simulink model "AE432_FinDel_Pioneer_WayPoint_Sim_2018a"  (R2018a)
settings: Solver=VariableStepAuto  StartTime=0  StopTime=445  FixedStep=T  RelTol=1e-3  EnableMultiTasking=on
InitFcn:
  | Waypoints
  | RollPitchTracking_Stab_ControlPioneer
values from neighbouring files (symbols this model uses):
  h = 220*ones(1,36)    [Waypoints.m]
  K1 = place(Along,Blong,P1)    [RollPitchTracking_Stab_ControlPioneer.m]
  T = 0.05    [Waypoints.m]
  x = [0 250 250 250 250 250 1250 2250 2150 2100 2050 2000 1900 1250 1250 500 500 500 500 1500 2250 2250 2250 2250 1000 1000 1000 1000 1250 1250 1250 1250 1750 1750 1750 1750]    [Waypoints.m]
  y = [0 1250 1750 2750 3500 4250 4250 4250 3750 3000 1750 1250 250 250 1500 2500 3000 3500 4000 4000 4000 3500 3000 2500 2500 3000 3500 4000 4000 3500 3000 2500 2500 3000 3500 4000]    [Waypoints.m]
undefined symbols (not defined in the file or in its folder): DiscIntNeverNeededParam, Td
libraries: simulink x19, simulink_extras x10, aerolibfltsims x2, airlib x1, aerolibanimutils x1
(part 2 of 2)

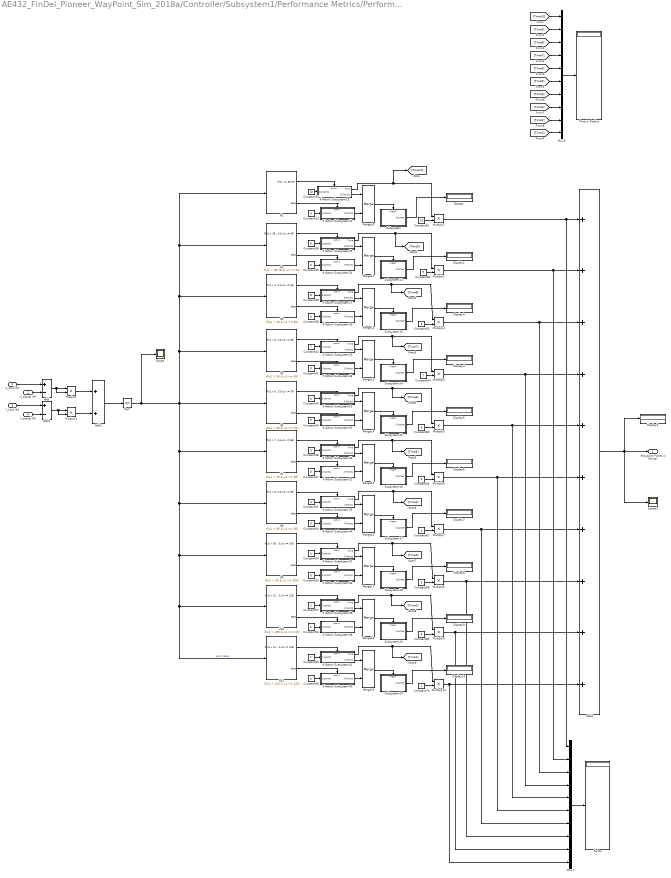
== system AE432_FinDel_Pioneer_WayPoint_Sim_2018a/Controller/Subsystem1/Performance Metrics/Performance Index Waypoints ==
  X_cmd (ft) : Inport
  X_actual (ft) : Inport  Port=2
  Y_cmd (ft) : Inport  Port=3
  Y_actual (ft) : Inport  Port=4
  Add : Sum  Inputs=+-
  Add1 : Sum  Inputs=+-
  Add2 : Sum
  Add4 : Sum  Inputs=10
  Constant{32,35,38,41,44,47,50,53,56,59} (10 alike) : Constant  Value=0
  Constant33 : Constant  Value=10
  Constant36 : Constant  Value=9
  Constant39 : Constant  Value=8
  Constant42 : Constant  Value=7
  Constant45 : Constant  Value=6
  Constant48 : Constant  Value=5
  Constant51 : Constant  Value=4
  Constant54 : Constant  Value=3
  Constant57 : Constant  Value=2
  Constant60 : Constant
  Constant61 : Constant  Value=10
  Constant62 : Constant  Value=9
  Constant63 : Constant  Value=8
  Constant64 : Constant  Value=7
  Constant65 : Constant  Value=6
  Constant66 : Constant  Value=5
  Constant67 : Constant  Value=4
  Constant68 : Constant  Value=3
  Constant69 : Constant  Value=2
  Constant70 : Constant
  Display{,1..10} (11 alike) : Display
  If Action Subsystem22 : Subsystem  TreatAsAtomicUnit=on
  If Action Subsystem23 : Subsystem  TreatAsAtomicUnit=on
  If Action Subsystem24 : Subsystem  TreatAsAtomicUnit=on
  If Action Subsystem25 : Subsystem  TreatAsAtomicUnit=on
  If Action Subsystem26 : Subsystem  TreatAsAtomicUnit=on
  If Action Subsystem27 : Subsystem  TreatAsAtomicUnit=on
  If Action Subsystem28 : Subsystem  TreatAsAtomicUnit=on
  If Action Subsystem29 : Subsystem  TreatAsAtomicUnit=on
  If Action Subsystem30 : Subsystem  TreatAsAtomicUnit=on
  If Action Subsystem31 : Subsystem  TreatAsAtomicUnit=on
  If Action Subsystem32 : Subsystem  TreatAsAtomicUnit=on
  If Action Subsystem33 : Subsystem  TreatAsAtomicUnit=on
  If Action Subsystem34 : Subsystem  TreatAsAtomicUnit=on
  If Action Subsystem35 : Subsystem  TreatAsAtomicUnit=on
  If Action Subsystem36 : Subsystem  TreatAsAtomicUnit=on
  If Action Subsystem37 : Subsystem  TreatAsAtomicUnit=on
  If Action Subsystem38 : Subsystem  TreatAsAtomicUnit=on
  If Action Subsystem39 : Subsystem  TreatAsAtomicUnit=on
  If Action Subsystem40 : Subsystem  TreatAsAtomicUnit=on
  If Action Subsystem41 : Subsystem  TreatAsAtomicUnit=on
  If10 : If  IfExpression=u1 > 105 & u1 <= 115
  If11 : If  IfExpression=u1 > 115 & u1 <= 125
  If2 : If  IfExpression=u1 <= 33.76
  If3 : If  IfExpression=u1 > 33.76 & u1 <= 45
  If4 : If  IfExpression=u1 > 45 & u1 <= 55
  If5 : If  IfExpression=u1 > 55 & u1 <= 65
  If6 : If  IfExpression=u1 > 65 & u1 <= 75
  If7 : If  IfExpression=u1 > 75 & u1 <= 85
  If8 : If  IfExpression=u1 > 85 & u1 <= 95
  If9 : If  IfExpression=u1 > 95 & u1 <= 105
  Merge{10..19} (10 alike) : Merge
  Multiply{1..10} (10 alike) : Product
  Mux1 : Mux  Inputs=10
  Mux2 : Mux  Inputs=10
  Points : Display
  Product : Product  RndMeth=Zero
  Product1 : Product  RndMeth=Zero
  Scope : Scope
  Scope2 : Scope
  Sqrt : Sqrt  SaturateOnIntegerOverflow=on
  Subsystem : Subsystem
  Subsystem12 : Subsystem
  Subsystem13 : Subsystem
  Subsystem14 : Subsystem
  Subsystem15 : Subsystem
  Subsystem16 : Subsystem
  Subsystem17 : Subsystem
  Subsystem18 : Subsystem
  Subsystem19 : Subsystem
  Subsystem20 : Subsystem
  Time in Radius : Display
  Waypoint Points = f(time) : Outport
  wires:
  Subsystem19/1(Counter) -> Display9/1
  Subsystem20/1(Counter) -> Display10/1
  Add/1 -> Product/2, Product/1
  Add1/1 -> Product1/2, Product1/1
  Y_actual (ft)/1 -> Add1/2
  Product1/1 -> Add2/2
  X_cmd (ft)/1 -> Add/1
  Product/1 -> Add2/1
  Y_cmd (ft)/1 -> Add1/1
  X_actual (ft)/1 -> Add/2
  Add2/1 -> Sqrt/1
  Sqrt/1 -> Scope/1, If11/1, If10/1, If9/1, If8/1, If7/1, If6/1, If5/1, If4/1, If3/1, If2/1  "error radius"
  If Action Subsystem22/1(0 Points) -> Merge10/2
  If Action Subsystem23/2(10 Points) -> Merge10/1
  Merge10/1 -> Subsystem/Trigger
  If2/1 -> If Action Subsystem23/Action
  Constant32/1 -> If Action Subsystem22/1("0 points  ")
  Constant33/1 -> If Action Subsystem23/1("10 points  ")
  If2/2 -> If Action Subsystem22/Action
  If3/2 -> If Action Subsystem24/Action
  Constant36/1 -> If Action Subsystem25/1("9 points  ")
  Constant35/1 -> If Action Subsystem24/1("0 points  ")
  If3/1 -> If Action Subsystem25/Action
  Merge11/1 -> Subsystem12/Trigger
  If Action Subsystem25/2(9 Points) -> Merge11/1
  If Action Subsystem24/1(0 Points) -> Merge11/2
  If Action Subsystem26/1(0 Points) -> Merge12/2
  If Action Subsystem27/2(8 Points) -> Merge12/1
  Merge12/1 -> Subsystem13/Trigger
  If4/1 -> If Action Subsystem27/Action
  Constant38/1 -> If Action Subsystem26/1("0 points  ")
  Constant39/1 -> If Action Subsystem27/1("8 points  ")
  If4/2 -> If Action Subsystem26/Action
  If5/2 -> If Action Subsystem28/Action
  Constant42/1 -> If Action Subsystem29/1("7 points  ")
  Constant41/1 -> If Action Subsystem28/1("0 points  ")
  If5/1 -> If Action Subsystem29/Action
  Merge13/1 -> Subsystem14/Trigger
  If Action Subsystem29/2(7 Points) -> Merge13/1
  If Action Subsystem28/1(0 Points) -> Merge13/2
  If Action Subsystem30/1(0 Points) -> Merge14/2
  If Action Subsystem31/2(6 Points) -> Merge14/1
  Merge14/1 -> Subsystem15/Trigger
  If6/1 -> If Action Subsystem31/Action
  Constant44/1 -> If Action Subsystem30/1("0 points  ")
  Constant45/1 -> If Action Subsystem31/1("6 points  ")
  If6/2 -> If Action Subsystem30/Action
  If7/2 -> If Action Subsystem32/Action
  Constant48/1 -> If Action Subsystem33/1("5 points  ")
  Constant47/1 -> If Action Subsystem32/1("0 points  ")
  If7/1 -> If Action Subsystem33/Action
  Merge15/1 -> Subsystem16/Trigger
  If Action Subsystem33/2(5 Points) -> Merge15/1
  If Action Subsystem32/1(0 Points) -> Merge15/2
  If Action Subsystem34/1(0 Points) -> Merge16/2
  If Action Subsystem35/2(4 Points) -> Merge16/1
  Merge16/1 -> Subsystem17/Trigger
  If8/1 -> If Action Subsystem35/Action
  Constant50/1 -> If Action Subsystem34/1("0 points  ")
  Constant51/1 -> If Action Subsystem35/1("4 points  ")
  If8/2 -> If Action Subsystem34/Action
  If9/2 -> If Action Subsystem36/Action
  Constant54/1 -> If Action Subsystem37/1("3 points  ")
  Constant53/1 -> If Action Subsystem36/1("0 points  ")
  If9/1 -> If Action Subsystem37/Action
  Merge17/1 -> Subsystem18/Trigger
  If Action Subsystem37/2(3 Points) -> Merge17/1
  If Action Subsystem36/1(0 Points) -> Merge17/2
  If Action Subsystem38/1(0 Points) -> Merge18/2
  If Action Subsystem39/2(2 Points) -> Merge18/1
  Merge18/1 -> Subsystem19/Trigger
  Constant56/1 -> If Action Subsystem38/1("0 points  ")
  Constant57/1 -> If Action Subsystem39/1("2 points  ")
  If10/2 -> If Action Subsystem38/Action
  If11/2 -> If Action Subsystem40/Action
  Constant60/1 -> If Action Subsystem41/1("1 points  ")
  Constant59/1 -> If Action Subsystem40/1("0 points  ")
  Merge19/1 -> Subsystem20/Trigger
  If Action Subsystem41/2(1 Points) -> Merge19/1
  If Action Subsystem40/1(0 Points) -> Merge19/2
  If10/1 -> If Action Subsystem39/Action
  If11/1 -> If Action Subsystem41/Action
  Subsystem/1(Counter) -> Display/1
  Subsystem12/1(Counter) -> Display1/1
  Subsystem13/1(Counter) -> Display3/1
  Subsystem14/1(Counter) -> Display4/1
  Subsystem15/1(Counter) -> Display5/1
  Subsystem16/1(Counter) -> Display6/1
  Subsystem17/1(Counter) -> Display7/1
  Subsystem18/1(Counter) -> Display8/1
  Multiply1/1 -> Mux1/1, Add4/1
  Multiply2/1 -> Mux1/2, Add4/2
  Multiply3/1 -> Mux1/3, Add4/3
  Multiply4/1 -> Mux1/4, Add4/4
  Multiply5/1 -> Mux1/5, Add4/5
  Multiply6/1 -> Mux1/6, Add4/6
  Multiply7/1 -> Mux1/7, Add4/7
  Multiply8/1 -> Mux1/8, Add4/8
  Multiply9/1 -> Mux1/9, Add4/9
  Multiply10/1 -> Mux1/10, Add4/10
  Mux1/1 -> Points/1
  Add4/1 -> Scope2/1, Waypoint Points = f(time)/1, Display2/1
  Constant61/1 -> Multiply1/2
  If Action Subsystem23/1(Time) -> [Time10], Multiply1/1
  Constant62/1 -> Multiply2/2
  If Action Subsystem25/1(Time) -> [Time9], Multiply2/1
  Constant63/1 -> Multiply3/2
  Constant64/1 -> Multiply4/2
  If Action Subsystem29/1(Time) -> [Time7], Multiply4/1
  Constant65/1 -> Multiply5/2
  If Action Subsystem31/1(Time) -> [Time6], Multiply5/1
  Constant66/1 -> Multiply6/2
  If Action Subsystem33/1(Time) -> [Time5], Multiply6/1
  Constant67/1 -> Multiply7/2
  If Action Subsystem35/1(Time) -> [Time4], Multiply7/1
  Constant68/1 -> Multiply8/2
  If Action Subsystem37/1(Time) -> [Time3], Multiply8/1
  Constant69/1 -> Multiply9/2
  If Action Subsystem39/1(Time) -> [Time2], Multiply9/1
  Constant70/1 -> Multiply10/2
  If Action Subsystem41/1(Time) -> [Time1], Multiply10/1
  Mux2/1 -> Time in Radius/1
  If Action Subsystem27/1(Time) -> [Time8], Multiply3/1
  [Time10] -> Mux2/1
  [Time9] -> Mux2/2
  [Time8] -> Mux2/3
  [Time7] -> Mux2/4
  [Time6] -> Mux2/5
  [Time5] -> Mux2/6
  [Time4] -> Mux2/7
  [Time3] -> Mux2/8
  [Time2] -> Mux2/9
  [Time1] -> Mux2/10

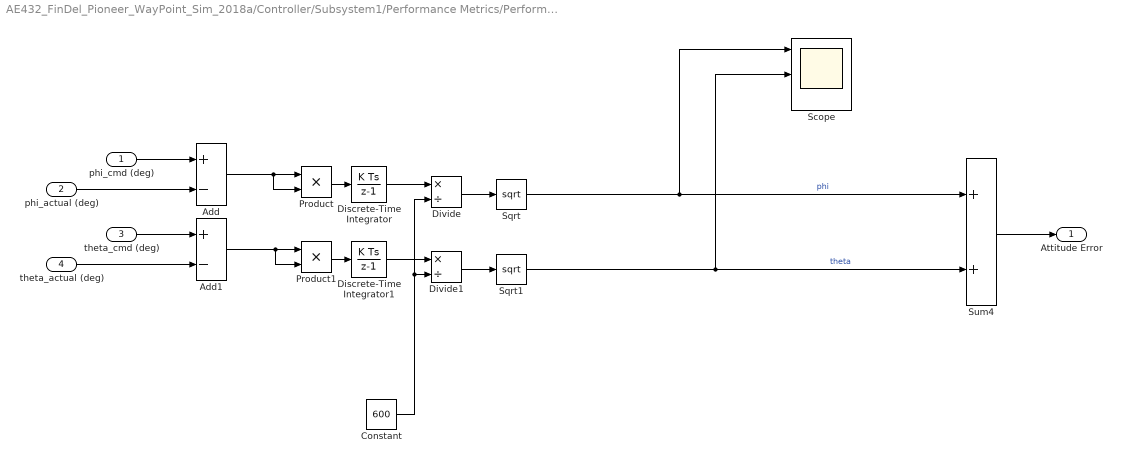
== system AE432_FinDel_Pioneer_WayPoint_Sim_2018a/Controller/Subsystem1/Performance Metrics/Performance Metric Attitude ==
  phi_cmd (deg) : Inport
  phi_actual (deg) : Inport  Port=2
  theta_cmd (deg) : Inport  Port=3
  theta_actual (deg) : Inport  Port=4
  Add : Sum  Inputs=+-
  Add1 : Sum  Inputs=+-
  Constant : Constant  Value=600
  Discrete-Time Integrator : DiscreteIntegrator  SampleTime=-1  ICPrevOutput=DiscIntNeverNeededParam  ICPrevScaledInput=DiscIntNeverNeededParam
  Discrete-Time Integrator1 : DiscreteIntegrator  SampleTime=-1  ICPrevOutput=DiscIntNeverNeededParam  ICPrevScaledInput=DiscIntNeverNeededParam
  Divide : Product  Inputs=*/
  Divide1 : Product  Inputs=*/
  Product : Product  RndMeth=Zero
  Product1 : Product  RndMeth=Zero
  Scope : Scope  NumInputPorts=3
  Sqrt : Sqrt  SaturateOnIntegerOverflow=on
  Sqrt1 : Sqrt  SaturateOnIntegerOverflow=on
  Sum4 : Sum
  Attitude Error : Outport
  wires:
  Constant/1 -> Divide/2, Divide1/2
  Discrete-Time Integrator1/1 -> Divide1/1
  Divide1/1 -> Sqrt1/1
  Product1/1 -> Discrete-Time Integrator1/1
  Discrete-Time Integrator/1 -> Divide/1
  Divide/1 -> Sqrt/1
  Product/1 -> Discrete-Time Integrator/1
  Sqrt1/1 -> Scope/2, Sum4/2  "theta"
  Sqrt/1 -> Scope/1, Sum4/1  "phi"
  Add/1 -> Product/2, Product/1
  Add1/1 -> Product1/2, Product1/1
  phi_cmd (deg)/1 -> Add/1
  phi_actual (deg)/1 -> Add/2
  theta_cmd (deg)/1 -> Add1/1
  theta_actual (deg)/1 -> Add1/2
  Sum4/1 -> Attitude Error/1

== system AE432_FinDel_Pioneer_WayPoint_Sim_2018a/Controller/Subsystem1/Performance Metrics/Outside Geo-fence/If Action Subsystem10 ==
  "0 points  " : Inport
  Action Port : ActionPort  InitializeStates=reset  ActionType=else
  0 Points : Outport
  wires:
  "0 points  "/1 -> 0 Points/1

== system AE432_FinDel_Pioneer_WayPoint_Sim_2018a/Controller/Subsystem1/Performance Metrics/Outside Geo-fence/If Action Subsystem5 ==
  "5 points  " : Inport
  Action Port : ActionPort  ActionType=then
  Add : Sum
  Constant2 : Constant  Value=0.05
  Delay1 : Delay  DelayLength=1  InitialCondition=0
  Time : Outport
  5 Points : Outport  Port=2
  wires:
  "5 points  "/1 -> 5 Points/1
  Constant2/1 -> Add/1
  Delay1/1 -> Add/2
  Add/1 -> Time/1, Delay1/1

== system AE432_FinDel_Pioneer_WayPoint_Sim_2018a/Controller/Subsystem1/Performance Metrics/Outside Geo-fence/Subsystem ==
  Trigger : TriggerPort  VariantControl=Variant  PortDimensions=1
  Add : Sum
  Constant2 : Constant  Value=0
  Delay1 : Delay  DelayLength=1  InitialCondition=0
  Increment Stored Integer : simulink/Additional Math & Discrete/Additional Math: Increment - Decrement/Increment Stored Integer
      settings: SourceProductName=Simulink
  Counter : Outport
  wires:
  Add/1 -> Increment Stored Integer/1
  Constant2/1 -> Add/1
  Delay1/1 -> Add/2
  Increment Stored Integer/1 -> Counter/1, Delay1/1

== system AE432_FinDel_Pioneer_WayPoint_Sim_2018a/Controller/Subsystem1/Performance Metrics/Performance Index Waypoints/If Action Subsystem22 ==
  "0 points  " : Inport
  Action Port : ActionPort  InitializeStates=reset  ActionType=else
  0 Points : Outport
  wires:
  "0 points  "/1 -> 0 Points/1

== system AE432_FinDel_Pioneer_WayPoint_Sim_2018a/Controller/Subsystem1/Performance Metrics/Performance Index Waypoints/If Action Subsystem23 ==
  "10 points  " : Inport
  Action Port : ActionPort  ActionType=then
  Add : Sum
  Constant2 : Constant  Value=0.05
  Delay1 : Delay  DelayLength=1  InitialCondition=0
  Time : Outport
  10 Points : Outport  Port=2
  wires:
  "10 points  "/1 -> 10 Points/1
  Constant2/1 -> Add/1
  Delay1/1 -> Add/2
  Add/1 -> Time/1, Delay1/1

== system AE432_FinDel_Pioneer_WayPoint_Sim_2018a/Controller/Subsystem1/Performance Metrics/Performance Index Waypoints/If Action Subsystem24 ==
  "0 points  " : Inport
  Action Port : ActionPort  InitializeStates=reset  ActionType=else
  0 Points : Outport
  wires:
  "0 points  "/1 -> 0 Points/1

== system AE432_FinDel_Pioneer_WayPoint_Sim_2018a/Controller/Subsystem1/Performance Metrics/Performance Index Waypoints/If Action Subsystem25 ==
  "9 points  " : Inport
  Action Port : ActionPort  ActionType=then
  Add : Sum
  Constant2 : Constant  Value=0.05
  Delay1 : Delay  DelayLength=1  InitialCondition=0
  Time : Outport
  9 Points : Outport  Port=2
  wires:
  "9 points  "/1 -> 9 Points/1
  Constant2/1 -> Add/1
  Delay1/1 -> Add/2
  Add/1 -> Time/1, Delay1/1

== system AE432_FinDel_Pioneer_WayPoint_Sim_2018a/Controller/Subsystem1/Performance Metrics/Performance Index Waypoints/If Action Subsystem26 ==
  "0 points  " : Inport
  Action Port : ActionPort  InitializeStates=reset  ActionType=else
  0 Points : Outport
  wires:
  "0 points  "/1 -> 0 Points/1

== system AE432_FinDel_Pioneer_WayPoint_Sim_2018a/Controller/Subsystem1/Performance Metrics/Performance Index Waypoints/If Action Subsystem27 ==
  "8 points  " : Inport
  Action Port : ActionPort  ActionType=then
  Add : Sum
  Constant2 : Constant  Value=0.05
  Delay1 : Delay  DelayLength=1  InitialCondition=0
  Time : Outport
  8 Points : Outport  Port=2
  wires:
  "8 points  "/1 -> 8 Points/1
  Constant2/1 -> Add/1
  Delay1/1 -> Add/2
  Add/1 -> Time/1, Delay1/1

== system AE432_FinDel_Pioneer_WayPoint_Sim_2018a/Controller/Subsystem1/Performance Metrics/Performance Index Waypoints/If Action Subsystem28 ==
  "0 points  " : Inport
  Action Port : ActionPort  InitializeStates=reset  ActionType=else
  0 Points : Outport
  wires:
  "0 points  "/1 -> 0 Points/1

== system AE432_FinDel_Pioneer_WayPoint_Sim_2018a/Controller/Subsystem1/Performance Metrics/Performance Index Waypoints/If Action Subsystem29 ==
  "7 points  " : Inport
  Action Port : ActionPort  ActionType=then
  Add : Sum
  Constant2 : Constant  Value=0.05
  Delay1 : Delay  DelayLength=1  InitialCondition=0
  Time : Outport
  7 Points : Outport  Port=2
  wires:
  "7 points  "/1 -> 7 Points/1
  Constant2/1 -> Add/1
  Delay1/1 -> Add/2
  Add/1 -> Time/1, Delay1/1

== system AE432_FinDel_Pioneer_WayPoint_Sim_2018a/Controller/Subsystem1/Performance Metrics/Performance Index Waypoints/If Action Subsystem30 ==
  "0 points  " : Inport
  Action Port : ActionPort  InitializeStates=reset  ActionType=else
  0 Points : Outport
  wires:
  "0 points  "/1 -> 0 Points/1

== system AE432_FinDel_Pioneer_WayPoint_Sim_2018a/Controller/Subsystem1/Performance Metrics/Performance Index Waypoints/If Action Subsystem31 ==
  "6 points  " : Inport
  Action Port : ActionPort  ActionType=then
  Add : Sum
  Constant2 : Constant  Value=0.05
  Delay1 : Delay  DelayLength=1  InitialCondition=0
  Time : Outport
  6 Points : Outport  Port=2
  wires:
  "6 points  "/1 -> 6 Points/1
  Constant2/1 -> Add/1
  Delay1/1 -> Add/2
  Add/1 -> Time/1, Delay1/1

== system AE432_FinDel_Pioneer_WayPoint_Sim_2018a/Controller/Subsystem1/Performance Metrics/Performance Index Waypoints/If Action Subsystem32 ==
  "0 points  " : Inport
  Action Port : ActionPort  InitializeStates=reset  ActionType=else
  0 Points : Outport
  wires:
  "0 points  "/1 -> 0 Points/1

== system AE432_FinDel_Pioneer_WayPoint_Sim_2018a/Controller/Subsystem1/Performance Metrics/Performance Index Waypoints/If Action Subsystem33 ==
  "5 points  " : Inport
  Action Port : ActionPort  ActionType=then
  Add : Sum
  Constant2 : Constant  Value=0.05
  Delay1 : Delay  DelayLength=1  InitialCondition=0
  Time : Outport
  5 Points : Outport  Port=2
  wires:
  "5 points  "/1 -> 5 Points/1
  Constant2/1 -> Add/1
  Delay1/1 -> Add/2
  Add/1 -> Time/1, Delay1/1

== system AE432_FinDel_Pioneer_WayPoint_Sim_2018a/Controller/Subsystem1/Performance Metrics/Performance Index Waypoints/If Action Subsystem34 ==
  "0 points  " : Inport
  Action Port : ActionPort  InitializeStates=reset  ActionType=else
  0 Points : Outport
  wires:
  "0 points  "/1 -> 0 Points/1

== system AE432_FinDel_Pioneer_WayPoint_Sim_2018a/Controller/Subsystem1/Performance Metrics/Performance Index Waypoints/If Action Subsystem35 ==
  "4 points  " : Inport
  Action Port : ActionPort  ActionType=then
  Add : Sum
  Constant2 : Constant  Value=0.05
  Delay1 : Delay  DelayLength=1  InitialCondition=0
  Time : Outport
  4 Points : Outport  Port=2
  wires:
  "4 points  "/1 -> 4 Points/1
  Constant2/1 -> Add/1
  Delay1/1 -> Add/2
  Add/1 -> Time/1, Delay1/1

== system AE432_FinDel_Pioneer_WayPoint_Sim_2018a/Controller/Subsystem1/Performance Metrics/Performance Index Waypoints/If Action Subsystem36 ==
  "0 points  " : Inport
  Action Port : ActionPort  InitializeStates=reset  ActionType=else
  0 Points : Outport
  wires:
  "0 points  "/1 -> 0 Points/1

== system AE432_FinDel_Pioneer_WayPoint_Sim_2018a/Controller/Subsystem1/Performance Metrics/Performance Index Waypoints/If Action Subsystem37 ==
  "3 points  " : Inport
  Action Port : ActionPort  ActionType=then
  Add : Sum
  Constant2 : Constant  Value=0.05
  Delay1 : Delay  DelayLength=1  InitialCondition=0
  Time : Outport
  3 Points : Outport  Port=2
  wires:
  "3 points  "/1 -> 3 Points/1
  Constant2/1 -> Add/1
  Delay1/1 -> Add/2
  Add/1 -> Time/1, Delay1/1

== system AE432_FinDel_Pioneer_WayPoint_Sim_2018a/Controller/Subsystem1/Performance Metrics/Performance Index Waypoints/If Action Subsystem38 ==
  "0 points  " : Inport
  Action Port : ActionPort  InitializeStates=reset  ActionType=else
  0 Points : Outport
  wires:
  "0 points  "/1 -> 0 Points/1

== system AE432_FinDel_Pioneer_WayPoint_Sim_2018a/Controller/Subsystem1/Performance Metrics/Performance Index Waypoints/If Action Subsystem39 ==
  "2 points  " : Inport
  Action Port : ActionPort  ActionType=then
  Add : Sum
  Constant2 : Constant  Value=0.05
  Delay1 : Delay  DelayLength=1  InitialCondition=0
  Time : Outport
  2 Points : Outport  Port=2
  wires:
  "2 points  "/1 -> 2 Points/1
  Constant2/1 -> Add/1
  Delay1/1 -> Add/2
  Add/1 -> Time/1, Delay1/1

== system AE432_FinDel_Pioneer_WayPoint_Sim_2018a/Controller/Subsystem1/Performance Metrics/Performance Index Waypoints/If Action Subsystem40 ==
  "0 points  " : Inport
  Action Port : ActionPort  InitializeStates=reset  ActionType=else
  0 Points : Outport
  wires:
  "0 points  "/1 -> 0 Points/1

== system AE432_FinDel_Pioneer_WayPoint_Sim_2018a/Controller/Subsystem1/Performance Metrics/Performance Index Waypoints/If Action Subsystem41 ==
  "1 points  " : Inport
  Action Port : ActionPort  ActionType=then
  Add : Sum
  Constant2 : Constant  Value=0.05
  Delay1 : Delay  DelayLength=1  InitialCondition=0
  Time : Outport
  1 Points : Outport  Port=2
  wires:
  "1 points  "/1 -> 1 Points/1
  Constant2/1 -> Add/1
  Delay1/1 -> Add/2
  Add/1 -> Time/1, Delay1/1

== system AE432_FinDel_Pioneer_WayPoint_Sim_2018a/Controller/Subsystem1/Performance Metrics/Performance Index Waypoints/Subsystem ==
  Trigger : TriggerPort  VariantControl=Variant  InitialTriggerSignalState=zero  PortDimensions=1
  Add : Sum
  Constant2 : Constant  Value=0
  Delay1 : Delay  DelayLength=1  InitialCondition=0
  Increment Stored Integer : simulink/Additional Math & Discrete/Additional Math: Increment - Decrement/Increment Stored Integer
      settings: SourceProductName=Simulink
  Counter : Outport
  wires:
  Add/1 -> Increment Stored Integer/1
  Constant2/1 -> Add/1
  Delay1/1 -> Add/2
  Increment Stored Integer/1 -> Counter/1, Delay1/1

== system AE432_FinDel_Pioneer_WayPoint_Sim_2018a/Controller/Subsystem1/Performance Metrics/Performance Index Waypoints/Subsystem12 ==
  Trigger : TriggerPort  VariantControl=Variant  InitialTriggerSignalState=zero  PortDimensions=1
  Add : Sum
  Constant2 : Constant  Value=0
  Delay1 : Delay  DelayLength=1  InitialCondition=0
  Increment Stored Integer : simulink/Additional Math & Discrete/Additional Math: Increment - Decrement/Increment Stored Integer
      settings: SourceProductName=Simulink
  Counter : Outport
  wires:
  Increment Stored Integer/1 -> Delay1/1, Counter/1
  Delay1/1 -> Add/2
  Constant2/1 -> Add/1
  Add/1 -> Increment Stored Integer/1

== system AE432_FinDel_Pioneer_WayPoint_Sim_2018a/Controller/Subsystem1/Performance Metrics/Performance Index Waypoints/Subsystem13 ==
  Trigger : TriggerPort  VariantControl=Variant  InitialTriggerSignalState=zero  PortDimensions=1
  Add : Sum
  Constant2 : Constant  Value=0
  Delay1 : Delay  DelayLength=1  InitialCondition=0
  Increment Stored Integer : simulink/Additional Math & Discrete/Additional Math: Increment - Decrement/Increment Stored Integer
      settings: SourceProductName=Simulink
  Counter : Outport
  wires:
  Add/1 -> Increment Stored Integer/1
  Constant2/1 -> Add/1
  Delay1/1 -> Add/2
  Increment Stored Integer/1 -> Counter/1, Delay1/1

== system AE432_FinDel_Pioneer_WayPoint_Sim_2018a/Controller/Subsystem1/Performance Metrics/Performance Index Waypoints/Subsystem14 ==
  Trigger : TriggerPort  VariantControl=Variant  InitialTriggerSignalState=zero  PortDimensions=1
  Add : Sum
  Constant2 : Constant  Value=0
  Delay1 : Delay  DelayLength=1  InitialCondition=0
  Increment Stored Integer : simulink/Additional Math & Discrete/Additional Math: Increment - Decrement/Increment Stored Integer
      settings: SourceProductName=Simulink
  Counter : Outport
  wires:
  Increment Stored Integer/1 -> Delay1/1, Counter/1
  Delay1/1 -> Add/2
  Constant2/1 -> Add/1
  Add/1 -> Increment Stored Integer/1

== system AE432_FinDel_Pioneer_WayPoint_Sim_2018a/Controller/Subsystem1/Performance Metrics/Performance Index Waypoints/Subsystem15 ==
  Trigger : TriggerPort  VariantControl=Variant  InitialTriggerSignalState=zero  PortDimensions=1
  Add : Sum
  Constant2 : Constant  Value=0
  Delay1 : Delay  DelayLength=1  InitialCondition=0
  Increment Stored Integer : simulink/Additional Math & Discrete/Additional Math: Increment - Decrement/Increment Stored Integer
      settings: SourceProductName=Simulink
  Counter : Outport
  wires:
  Add/1 -> Increment Stored Integer/1
  Constant2/1 -> Add/1
  Delay1/1 -> Add/2
  Increment Stored Integer/1 -> Counter/1, Delay1/1

== system AE432_FinDel_Pioneer_WayPoint_Sim_2018a/Controller/Subsystem1/Performance Metrics/Performance Index Waypoints/Subsystem16 ==
  Trigger : TriggerPort  VariantControl=Variant  InitialTriggerSignalState=zero  PortDimensions=1
  Add : Sum
  Constant2 : Constant  Value=0
  Delay1 : Delay  DelayLength=1  InitialCondition=0
  Increment Stored Integer : simulink/Additional Math & Discrete/Additional Math: Increment - Decrement/Increment Stored Integer
      settings: SourceProductName=Simulink
  Counter : Outport
  wires:
  Increment Stored Integer/1 -> Delay1/1, Counter/1
  Delay1/1 -> Add/2
  Constant2/1 -> Add/1
  Add/1 -> Increment Stored Integer/1

== system AE432_FinDel_Pioneer_WayPoint_Sim_2018a/Controller/Subsystem1/Performance Metrics/Performance Index Waypoints/Subsystem17 ==
  Trigger : TriggerPort  VariantControl=Variant  InitialTriggerSignalState=zero  PortDimensions=1
  Add : Sum
  Constant2 : Constant  Value=0
  Delay1 : Delay  DelayLength=1  InitialCondition=0
  Increment Stored Integer : simulink/Additional Math & Discrete/Additional Math: Increment - Decrement/Increment Stored Integer
      settings: SourceProductName=Simulink
  Counter : Outport
  wires:
  Add/1 -> Increment Stored Integer/1
  Constant2/1 -> Add/1
  Delay1/1 -> Add/2
  Increment Stored Integer/1 -> Counter/1, Delay1/1

== system AE432_FinDel_Pioneer_WayPoint_Sim_2018a/Controller/Subsystem1/Performance Metrics/Performance Index Waypoints/Subsystem18 ==
  Trigger : TriggerPort  VariantControl=Variant  InitialTriggerSignalState=zero  PortDimensions=1
  Add : Sum
  Constant2 : Constant  Value=0
  Delay1 : Delay  DelayLength=1  InitialCondition=0
  Increment Stored Integer : simulink/Additional Math & Discrete/Additional Math: Increment - Decrement/Increment Stored Integer
      settings: SourceProductName=Simulink
  Counter : Outport
  wires:
  Increment Stored Integer/1 -> Delay1/1, Counter/1
  Delay1/1 -> Add/2
  Constant2/1 -> Add/1
  Add/1 -> Increment Stored Integer/1

== system AE432_FinDel_Pioneer_WayPoint_Sim_2018a/Controller/Subsystem1/Performance Metrics/Performance Index Waypoints/Subsystem19 ==
  Trigger : TriggerPort  VariantControl=Variant  InitialTriggerSignalState=zero  PortDimensions=1
  Add : Sum
  Constant2 : Constant  Value=0
  Delay1 : Delay  DelayLength=1  InitialCondition=0
  Increment Stored Integer : simulink/Additional Math & Discrete/Additional Math: Increment - Decrement/Increment Stored Integer
      settings: SourceProductName=Simulink
  Counter : Outport
  wires:
  Add/1 -> Increment Stored Integer/1
  Constant2/1 -> Add/1
  Delay1/1 -> Add/2
  Increment Stored Integer/1 -> Counter/1, Delay1/1

== system AE432_FinDel_Pioneer_WayPoint_Sim_2018a/Controller/Subsystem1/Performance Metrics/Performance Index Waypoints/Subsystem20 ==
  Trigger : TriggerPort  VariantControl=Variant  InitialTriggerSignalState=zero  PortDimensions=1
  Add : Sum
  Constant2 : Constant  Value=0
  Delay1 : Delay  DelayLength=1  InitialCondition=0
  Increment Stored Integer : simulink/Additional Math & Discrete/Additional Math: Increment - Decrement/Increment Stored Integer
      settings: SourceProductName=Simulink
  Counter : Outport
  wires:
  Increment Stored Integer/1 -> Delay1/1, Counter/1
  Delay1/1 -> Add/2
  Constant2/1 -> Add/1
  Add/1 -> Increment Stored Integer/1
